simulink model "Model_2"  (R2025b)
settings: Solver=ode4  StartTime=0.0  StopTime=60  FixedStep=0.2  RelTol=1e-3
settings Model: Creator=danielborkovec  LastModifiedBy=danielborkovec

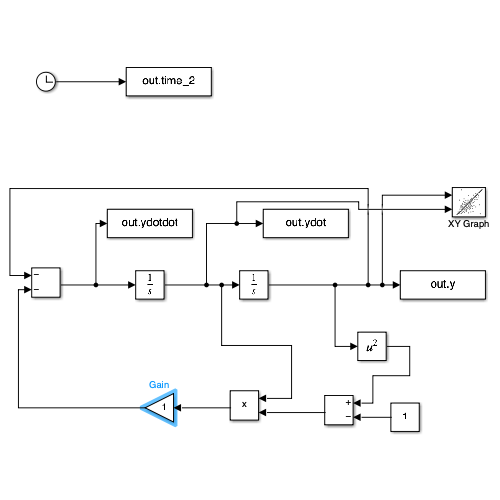
[thumbnail: Simulink's stored preview of the top-level diagram]
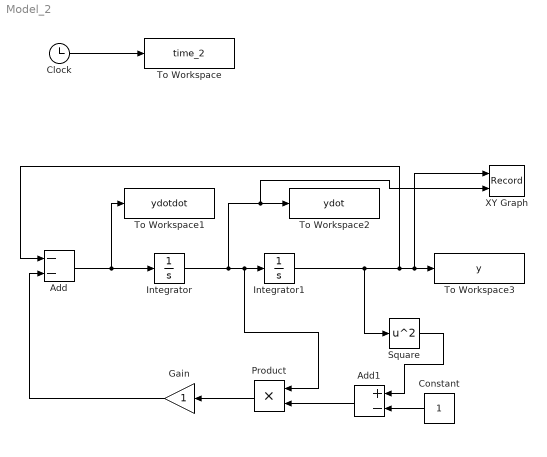
== system Model_2 ==
  Add : Sum  Inputs=--
  Add1 : Sum  Inputs=+-
  Clock : Clock
  Constant : Constant
  Gain : Gain
  Integrator : Integrator  InitialCondition=0.5
  Integrator1 : Integrator  InitialCondition=-0.5
  Product : Product
  Square : Math  Operator=square
  To Workspace : ToWorkspace  VariableName=time_2  SampleTime=-1
  To Workspace1 : ToWorkspace  VariableName=ydotdot  SampleTime=-1
  To Workspace2 : ToWorkspace  VariableName=ydot  SampleTime=-1
  To Workspace3 : ToWorkspace  VariableName=y  SampleTime=-1
  XY Graph : Record  NumPorts=2.0  FileSettingsInternal="{\"entries\":[{\"content\":{\"excelSettings\":{\"content\":{},\"type\":\"Streamout.ExcelSettings\"},\"parquetSettings\":{\"content\":{},\"type\":\"Streamout.ParquetSettings\"}},\"type\":\"Streamout.FileSettingStorage\",\"uuid\":\"\"}],\"packageUris\":[\"http:\\/\\/schema.mathworks.com\\/mf0\\/streamout_blocks\\/R2020a\"],\"version\":\"1.0\"}"  FrameSettings=[0, 0]  Layout=[1 1]  SignalsInternal="{\"entries\":[{\"content\":{\"signals\":[{\"content\":{\"blockPath\":[],\"dimensions\":[1],\"domain\":\"\",\"lineColor\":\"#a2142f\",\"plots\":[ 1 ],\"port\":1,\"sid\":[\"\"],\"signalID\":1,\"signalName\":\"Integrator1\"},\"type\":\"RecordBlkView.Signal\",\"uuid\":\"\"},{\"content\":{\"blockPath\":[],\"dimensions\":[1],\"domain\":\"\",\"lineColor\":\"#139fff\",\"plots\":[ 1 ],\"port\":2,\"sid\":[\"\"],\"signalID\":2,\"signalName\":\"Integrator\"},\"type\":\"RecordBlkView.Signal\",\"uuid\":\"\"}]},\"type\":\"RecordBlkView.InputSignals\",\"uuid\":\"\"}],\"packageUris\":[\"http:\\/\\/schema.mathworks.com\\/mf0\\/streamout_blocks\\/R2020a\"],\"version\":\"1.0\"}"  VisualizationBindings="{\"xyplotplugin\":{\"info\":[{\"series\":[{\"bindingParametersList\":[{\"parameter\":\"X-Axis\",\"signalID\":1,\"signalName\":\"Integrator1\"},{\"parameter\":\"Y-Axis\",\"signalID\":2,\"signalName\":\"Integrator\"}],\"seriesID\":0}],\"subplotID\":1}]}}"  CompatibilityTag=XY
  wires:
  Clock/1 -> To Workspace/1
  Add/1 -> To Workspace1/1, Integrator/1
  Integrator/1 -> XY Graph/2, To Workspace2/1, Product/1, Integrator1/1
  Product/1 -> Gain/1
  Gain/1 -> Add/2
  Constant/1 -> Add1/2
  Add1/1 -> Product/2
  Integrator1/1 -> Square/1, Add/1, XY Graph/1, To Workspace3/1
  Square/1 -> Add1/1
